simulink model "simTest"  (R2022b)
settings: Solver=VariableStepAuto  StartTime=0.0  StopTime=10.0  RelTol=1e-3
settings Model: Creator=AnasHamrouni  LastModifiedBy=AnasHamrouni

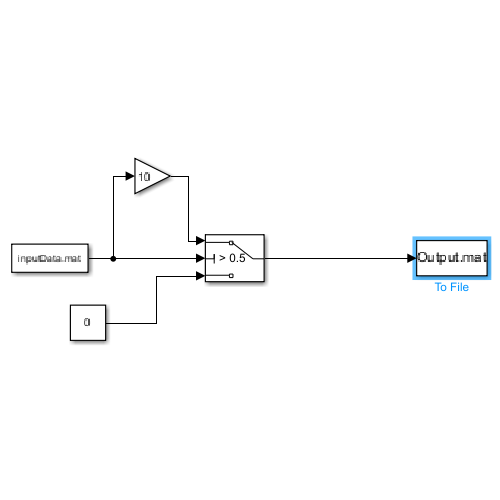
[thumbnail: Simulink's stored preview of the top-level diagram]
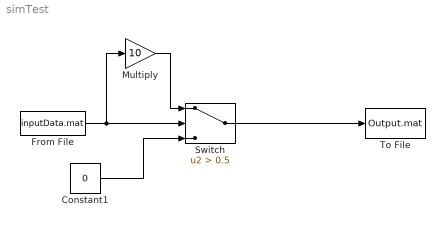
== system simTest ==
  Constant1 : Constant  Value=0
  From File : FromFile  FileName=inputData.mat  SampleTime=0
  Multiply : Gain  Gain=10
  Switch : Switch  Criteria=u2 > Threshold  Threshold=0.5  SaturateOnIntegerOverflow=off  InputSameDT=off
  To File : ToFile  Filename=Output.mat  SaveFormat=Timeseries
  wires:
  From File/1 -> Multiply/1, Switch/2
  Constant1/1 -> Switch/3
  Multiply/1 -> Switch/1
  Switch/1 -> To File/1
